simulink model "ComtradeRec_v2"  (R2017a)
settings: Solver=VariableStepAuto  StartTime=0.0  StopTime=0.15  MaxStep=1e-4  RelTol=1e-3
undefined symbols (not defined in the file or in its folder): D11, Delta
libraries: powerlib x27, powerlib_meascontrol x2
settings Model: Creator=Alexander  LastModifiedBy=Alexander
settings DataIOCC: SaveFormat=Array
settings DebuggingCC: MaxConsecutiveZCsMsg=none

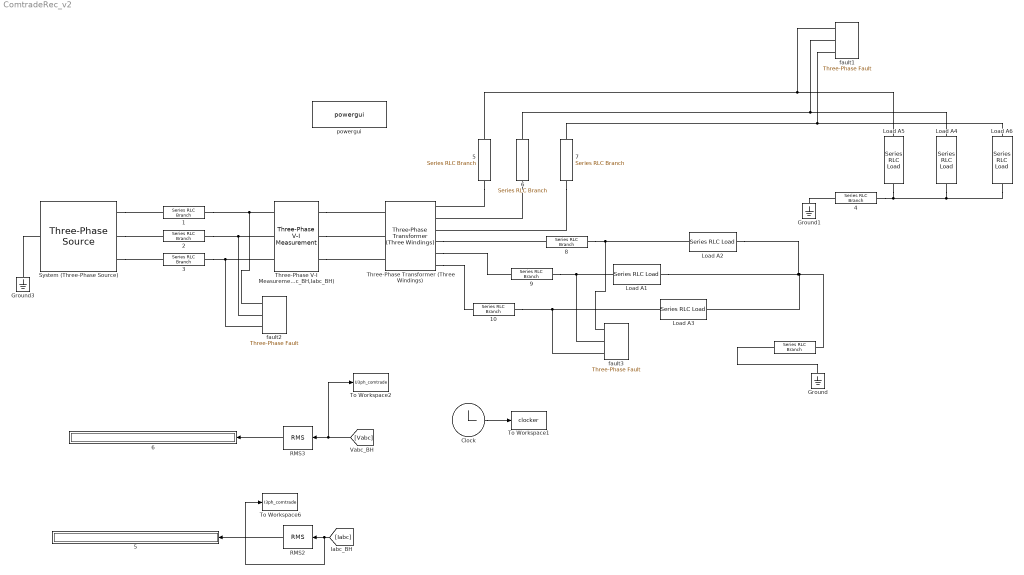
== system ComtradeRec_v2 ==
  " " : powerlib/Elements/Series RLC Branch  LConnTagsString=__new0  RConnTagsString=__new0  BranchType=RL  Resistance=0.001  Inductance=0.00006  SetiL0=off  InitialCurrent=0  Capacitance=1e-6  Setx0=off  InitialVoltage=0  Measurements=None
   {1..3,5..10} (9 alike) : powerlib/Elements/Series RLC Branch  LConnTagsString=__new0  RConnTagsString=__new0  BranchType=RLC  Resistance=1  Inductance=0.6  SetiL0=off  InitialCurrent=0  Capacitance=10e-6  Setx0=off  InitialVoltage=0  Measurements=None
  " 4" : powerlib/Elements/Series RLC Branch  LConnTagsString=__new0  RConnTagsString=__new0  BranchType=RL  Resistance=0.001  Inductance=0.00006  SetiL0=off  InitialCurrent=0  Capacitance=1e-6  Setx0=off  InitialVoltage=0  Measurements=None
  " 5" : Display
  " 6" : Display
  Clock : Clock
  Ground : powerlib/Elements/Ground  LConnTagsString=a
  Ground1 : powerlib/Elements/Ground  LConnTagsString=a
  Ground3 : powerlib/Elements/Ground  LConnTagsString=a
  Load A1 : powerlib/Elements/Series RLC Load  LConnTagsString=a  RConnTagsString=__new0  NominalVoltage=220000  NominalFrequency=50  ActivePower=400637.8312  InductivePower=415000  CapacitivePower=0  Setx0=off  InitialVoltage=0  SetiL0=off  InitialCurrent=0  Measurements=Branch voltage and current  LoadType=constant Z
  Load A2 : powerlib/Elements/Series RLC Load  LConnTagsString=a  RConnTagsString=__new0  NominalVoltage=110000  NominalFrequency=50  ActivePower=406113.3519  InductivePower=415000  CapacitivePower=0  Setx0=off  InitialVoltage=0  SetiL0=off  InitialCurrent=0  Measurements=Branch voltage and current  LoadType=constant Z
  Load A3 : powerlib/Elements/Series RLC Load  LConnTagsString=a  RConnTagsString=__new0  NominalVoltage=110000  NominalFrequency=50  ActivePower=401093.1769  InductivePower=415000  CapacitivePower=0  Setx0=off  InitialVoltage=0  SetiL0=off  InitialCurrent=0  Measurements=Branch voltage and current  LoadType=constant Z
  Load A4 : powerlib/Elements/Series RLC Load  LConnTagsString=a  RConnTagsString=__new0  NominalVoltage=220000  NominalFrequency=50  ActivePower=229.8979  InductivePower=415000  CapacitivePower=0  Setx0=off  InitialVoltage=0  SetiL0=off  InitialCurrent=0  Measurements=Branch voltage and current  LoadType=constant Z
  Load A5 : powerlib/Elements/Series RLC Load  LConnTagsString=a  RConnTagsString=__new0  NominalVoltage=110000  NominalFrequency=50  ActivePower=601310.9772  InductivePower=415000  CapacitivePower=0  Setx0=off  InitialVoltage=0  SetiL0=off  InitialCurrent=0  Measurements=Branch voltage and current  LoadType=constant Z
  Load A6 : powerlib/Elements/Series RLC Load  LConnTagsString=a  RConnTagsString=__new0  NominalVoltage=110000  NominalFrequency=50  ActivePower=608752.0618  InductivePower=415000  CapacitivePower=0  Setx0=off  InitialVoltage=0  SetiL0=off  InitialCurrent=0  Measurements=Branch voltage and current  LoadType=constant Z
  RMS2 : powerlib_meascontrol/Measurements/RMS  TrueRMS=on  Freq=50  RMSInit=0  Ts=0
  RMS3 : powerlib_meascontrol/Measurements/RMS  TrueRMS=on  Freq=50  RMSInit=0  Ts=0
  System (Three-Phase Source) : powerlib/Electrical Sources/Three-Phase Source  InternalConnection=Yn  VoltagePhases=off  Voltage=220e3  PhaseAngle=0  Voltage_phases=[25e3 25e3 25e3]/sqrt(3)  PhaseAngles_phases=[0 -120 +120]  Frequency=50  NonIdealSource=on  SpecifyImpedance=off  Resistance=5  Inductance=0  ShortCircuitLevel=100e6  BaseVoltage=220e3  XRratio=7  BusType=swing  Pref=10e3  Qref=0  Prefabc=[10e3, 10e3, 10e3]  Qrefabc=[0, 0, 0]  Qmin=-inf  Qmax=inf
  Three-Phase Transformer (Three Windings) : powerlib/Elements/Three-Phase Transformer (Three Windings)  Winding1Connection=Yg  Winding2Connection=Delta (D11)  Winding3Connection=Delta (D11)  CoreType=Three single-phase transformers  SetSaturation=off  Hysteresis=off  DataFile='hysteresis'  SetInitialFlux=off  Measurements=None  UNITS=pu  NominalPower=[ 250e6 , 60 ]  Winding1=[ 220e3 , 0.002 , 0.08 ]  Winding2=[ 110e3 , 0.002 , 0.08 ]  Winding3=[ 35e3 , 0.002 , 0.08 ]  Rm=500  Lm=500  L0=0.5  Saturation=[ 0,0 ; 0.0024,1.2 ; 1.0,1.52 ]  InitialFluxes=[0.8 -0.8 0.7]  MoreParameters=off  BreakLoop=off  DataType=off  TransfoNumber=1
      settings: SourceProductName=Simscape Power Systems  SourceProductBaseCode=PS
  Three-Phase V-I Measurement(Uabc_BH,Iabc_BH) : powerlib/Measurements/Three-Phase V-I Measurement  VoltageMeasurement=phase-to-ground  SetLabelV=on  LabelV=Vabc  Vpu=off  VpuLL=off  CurrentMeasurement=yes  SetLabelI=on  LabelI=Iabc  Ipu=off  Pbase=100e6  Vbase=500e3  OutputType=Complex  PhasorSimulation=off  PSBequivalent=0
  To Workspace1 : ToWorkspace  VariableName=clocker  SaveFormat=Timeseries  SampleTime=-1
  To Workspace2 : ToWorkspace  VariableName=U3ph_comtrade  SaveFormat=Structure With Time  SampleTime=-1
  To Workspace6 : ToWorkspace  VariableName=I3ph_comtrade  SaveFormat=Structure With Time  SampleTime=-1
  fault1 : powerlib/Elements/Three-Phase Fault  InitialStates=0  FaultA=off  FaultB=off  FaultC=off  GroundFault=on  SwitchTimes=[0.013635 0.023628]  External=off  SwitchStatus=NaN  FaultResistance=0.001  GroundResistance=0.01  SnubberResistance=1e6  SnubberCapacitance=inf  Measurements=None
  fault2 : powerlib/Elements/Three-Phase Fault  InitialStates=0  FaultA=off  FaultB=off  FaultC=off  GroundFault=off  SwitchTimes="[1/80  3/80]"  External=off  SwitchStatus=NaN  FaultResistance=0.001  GroundResistance=0.01  SnubberResistance=1e6  SnubberCapacitance=inf  Measurements=None
  fault3 : powerlib/Elements/Three-Phase Fault  InitialStates=0  FaultA=off  FaultB=off  FaultC=off  GroundFault=off  SwitchTimes="[1/80  3/80]"  External=off  SwitchStatus=NaN  FaultResistance=0.001  GroundResistance=0.01  SnubberResistance=1e6  SnubberCapacitance=inf  Measurements=None
  powergui : powerlib/powergui  Priority=1  SimulationMode=Continuous  SampleTime=50e-6  frequency=60  Iterations=50  frequencyindice=50  Pbase=100e6  ErrMax=1e-4  UnitsV=kV  UnitsW=MW  buscounter=0  FunctionMessages=off  echomessages=off  EnableUseOfTLC=off  CurrentSourceSwitches=off  DisableSnubberDevices=off  DisableRonSwitches=off  DisableVfSwitches=off  DisplayEquations=off  SolverType=Tustin/Backward Euler (TBE)  Interpol=off  ExternalGateDelay=off  methode=off  Ts=100  x0status=blocks  SPID=on  SwTol=0  HookPort=off  RestoreLinks=warning  ResistiveCurrentMeasurement=off  Frange=[0:2:500]  Ylog=off  Xlog=on  ShowGrid=off  save=off  variable=ZData  structure=0  ZoomFFT=off  StartTime=0.0  cycles=1  DisplayStyle=1  fundamental=60  FreqAxis=off  MaxFrequency=1000  frequencyindicesteady=1  RmsSteady=1  display=off
  wires:
  RMS3/1 -> " 6"/1
  Clock/1 -> To Workspace1/1
  [Vabc] -> To Workspace2/1, RMS3/1
  [Iabc] -> To Workspace6/1, RMS2/1
  RMS2/1 -> " 5"/1
  connections:
  System (Three-Phase Source)/RConn2 -- " 2"/LConn1
  " "/LConn1 -- Ground/LConn1
  System (Three-Phase Source)/LConn1 -- Ground3/LConn1
  Load A1/RConn1 -- Load A2/RConn1 -- " "/RConn1 -- Load A3/RConn1
  System (Three-Phase Source)/RConn1 -- " 1"/LConn1
  System (Three-Phase Source)/RConn3 -- " 3"/LConn1
  Load A6/RConn1 -- Load A4/RConn1 -- Load A5/RConn1 -- " 4"/RConn1
  " 4"/LConn1 -- Ground1/LConn1
  " 5"/RConn1 -- fault1/LConn1 -- Load A5/LConn1
  " 6"/RConn1 -- fault1/LConn2 -- Load A4/LConn1
  " 7"/RConn1 -- fault1/LConn3 -- Load A6/LConn1
  " 5"/LConn1 -- Three-Phase Transformer (Three Windings)/RConn1
  " 6"/LConn1 -- Three-Phase Transformer (Three Windings)/RConn2
  " 7"/LConn1 -- Three-Phase Transformer (Three Windings)/RConn3
  Three-Phase Transformer (Three Windings)/RConn4 -- " 8"/LConn1
  Three-Phase Transformer (Three Windings)/RConn5 -- " 9"/LConn1
  Three-Phase Transformer (Three Windings)/RConn6 -- " 10"/LConn1
  " 10"/RConn1 -- fault3/LConn3 -- Load A3/LConn1
  " 9"/RConn1 -- fault3/LConn2 -- Load A1/LConn1
  " 8"/RConn1 -- fault3/LConn1 -- Load A2/LConn1
  " 1"/RConn1 -- fault2/LConn1 -- Three-Phase V-I Measurement(Uabc_BH,Iabc_BH)/LConn1
  " 2"/RConn1 -- fault2/LConn2 -- Three-Phase V-I Measurement(Uabc_BH,Iabc_BH)/LConn2
  " 3"/RConn1 -- fault2/LConn3 -- Three-Phase V-I Measurement(Uabc_BH,Iabc_BH)/LConn3
  Three-Phase V-I Measurement(Uabc_BH,Iabc_BH)/RConn1 -- Three-Phase Transformer (Three Windings)/LConn1
  Three-Phase V-I Measurement(Uabc_BH,Iabc_BH)/RConn2 -- Three-Phase Transformer (Three Windings)/LConn2
  Three-Phase V-I Measurement(Uabc_BH,Iabc_BH)/RConn3 -- Three-Phase Transformer (Three Windings)/LConn3
